simulink model "case2mod"  (Simulink 7.7)
settings: Solver=FixedStepDiscrete  StartTime=0.0  StopTime=25000  FixedStep=1  RelTol=1e-3
libraries: SimpleModeling x38
settings Model: Creator=iris  LastModifiedBy=iris
settings DataIOCC: SaveFormat=StructureWithTime
settings OptimizationCC: BlockReduction=off  ConditionallyExecuteInputs=off

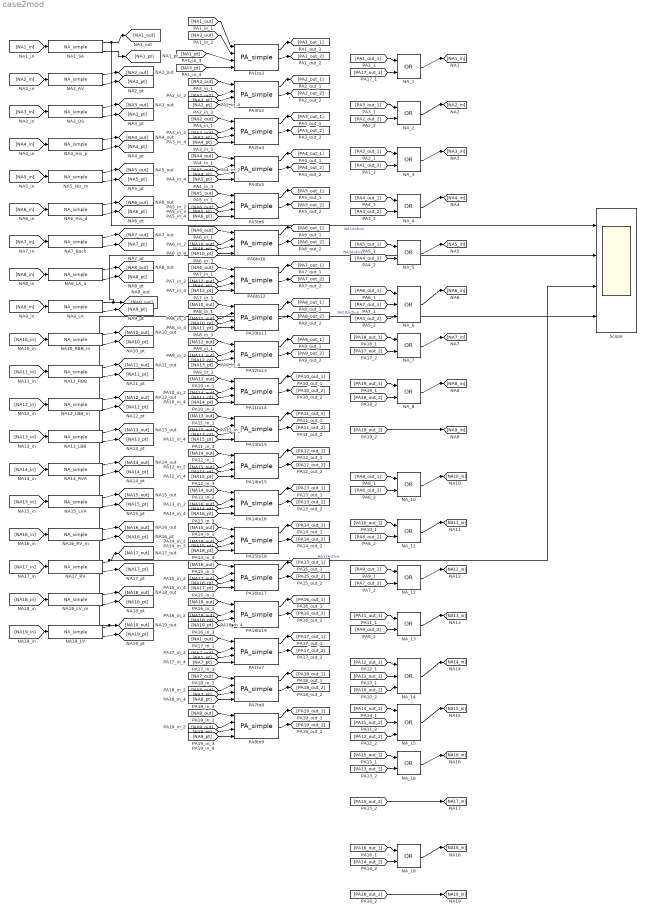
== system case2mod ==
  NA10_RBB_m : SimpleModeling/NA_simple  SystemSampleTime=-1  TERP_defs=320  TRRP_def=120  Trest_def=9999  TERP_s=320  TRRP_s=120  Trest_s=9999  Terp_min=150  Terp_max=300
  NA11_RBB : SimpleModeling/NA_simple  SystemSampleTime=-1  TERP_defs=320  TRRP_def=120  Trest_def=9999  TERP_s=320  TRRP_s=120  Trest_s=9999  Terp_min=150  Terp_max=300
  NA12_LBB_m : SimpleModeling/NA_simple  SystemSampleTime=-1  TERP_defs=320  TRRP_def=120  Trest_def=9999  TERP_s=320  TRRP_s=120  Trest_s=9999  Terp_min=150  Terp_max=300
  NA13_LBB : SimpleModeling/NA_simple  SystemSampleTime=-1  TERP_defs=320  TRRP_def=120  Trest_def=9999  TERP_s=320  TRRP_s=120  Trest_s=9999  Terp_min=150  Terp_max=300
  NA14_RVA : SimpleModeling/NA_simple  SystemSampleTime=-1  TERP_defs=320  TRRP_def=120  Trest_def=9999  TERP_s=320  TRRP_s=120  Trest_s=9999  Terp_min=150  Terp_max=300
  NA15_LVA : SimpleModeling/NA_simple  SystemSampleTime=-1  TERP_defs=320  TRRP_def=120  Trest_def=9999  TERP_s=320  TRRP_s=120  Trest_s=9999  Terp_min=150  Terp_max=300
  NA16_RV_m : SimpleModeling/NA_simple  SystemSampleTime=-1  TERP_defs=320  TRRP_def=120  Trest_def=9999  TERP_s=320  TRRP_s=120  Trest_s=9999  Terp_min=150  Terp_max=300
  NA17_RV : SimpleModeling/NA_simple  SystemSampleTime=-1  TERP_defs=320  TRRP_def=120  Trest_def=9999  TERP_s=320  TRRP_s=120  Trest_s=9999  Terp_min=150  Terp_max=300
  NA18_LV_m : SimpleModeling/NA_simple  SystemSampleTime=-1  TERP_defs=320  TRRP_def=120  Trest_def=9999  TERP_s=320  TRRP_s=120  Trest_s=9999  Terp_min=150  Terp_max=300
  NA19_LV : SimpleModeling/NA_simple  SystemSampleTime=-1  TERP_defs=320  TRRP_def=120  Trest_def=9999  TERP_s=320  TRRP_s=120  Trest_s=9999  Terp_min=150  Terp_max=300
  NA1_SA : SimpleModeling/NA_simple  SystemSampleTime=-1  TERP_defs=320  TRRP_def=100  Trest_def=800  TERP_s=320  TRRP_s=100  Trest_s=800  Terp_min=150  Terp_max=300
  NA2_AV : SimpleModeling/NA_simple  SystemSampleTime=-1  TERP_defs=320  TRRP_def=350  Trest_def=9999  TERP_s=320  TRRP_s=350  Trest_s=9999  Terp_min=800  Terp_max=350
  NA3_OS : SimpleModeling/NA_simple  SystemSampleTime=-1  TERP_defs=320  TRRP_def=120  Trest_def=9999  TERP_s=320  TRRP_s=120  Trest_s=9999  Terp_min=150  Terp_max=300
  NA4_His_p : SimpleModeling/NA_simple  SystemSampleTime=-1  TERP_defs=320  TRRP_def=120  Trest_def=9999  TERP_s=320  TRRP_s=120  Trest_s=9999  Terp_min=150  Terp_max=300
  NA5_His_m : SimpleModeling/NA_simple  SystemSampleTime=-1  TERP_defs=320  TRRP_def=120  Trest_def=9999  TERP_s=320  TRRP_s=120  Trest_s=9999  Terp_min=150  Terp_max=300
  NA6_His_d : SimpleModeling/NA_simple  SystemSampleTime=-1  TERP_defs=320  TRRP_def=120  Trest_def=9999  TERP_s=320  TRRP_s=120  Trest_s=9999  Terp_min=150  Terp_max=300
  NA7_Bach : SimpleModeling/NA_simple  SystemSampleTime=-1  TERP_defs=320  TRRP_def=120  Trest_def=9999  TERP_s=320  TRRP_s=120  Trest_s=9999  Terp_min=150  Terp_max=300
  NA8_LA_a : SimpleModeling/NA_simple  SystemSampleTime=-1  TERP_defs=320  TRRP_def=120  Trest_def=9999  TERP_s=320  TRRP_s=120  Trest_s=9999  Terp_min=150  Terp_max=300
  NA9_LA : SimpleModeling/NA_simple  SystemSampleTime=-1  TERP_defs=320  TRRP_def=120  Trest_def=9999  TERP_s=320  TRRP_s=120  Trest_s=9999  Terp_min=150  Terp_max=300
  NA_{1..5,7..8,10..13,16,18} (13 alike) : Logic  Operator=OR  AllPortsSameDT=off  OutDataTypeStr=boolean
  NA_14 : Logic  Operator=OR  Inputs=3  AllPortsSameDT=off  OutDataTypeStr=boolean
  NA_15 : Logic  Operator=OR  Inputs=3  AllPortsSameDT=off  OutDataTypeStr=boolean
  NA_6 : Logic  Operator=OR  Inputs=3  AllPortsSameDT=off  OutDataTypeStr=boolean
  PA10to11 : SimpleModeling/PA_simple  SystemSampleTime=-1  min_path_par=10  bck_param=43  forw_param=43
  PA11to14 : SimpleModeling/PA_simple  SystemSampleTime=-1  min_path_par=9  bck_param=9  forw_param=9
  PA12to13 : SimpleModeling/PA_simple  SystemSampleTime=-1  min_path_par=38  bck_param=38  forw_param=38
  PA13to15 : SimpleModeling/PA_simple  SystemSampleTime=-1  min_path_par=9  bck_param=10  forw_param=10
  PA14to15 : SimpleModeling/PA_simple  SystemSampleTime=-1  min_path_par=17  bck_param=18  forw_param=18
  PA14to16 : SimpleModeling/PA_simple  SystemSampleTime=-1  min_path_par=58  bck_param=58  forw_param=58
  PA15to18 : SimpleModeling/PA_simple  SystemSampleTime=-1  min_path_par=46  bck_param=46  forw_param=46
  PA16to17 : SimpleModeling/PA_simple  SystemSampleTime=-1  min_path_par=53  bck_param=53  forw_param=53
  PA18to19 : SimpleModeling/PA_simple  SystemSampleTime=-1  min_path_par=39  bck_param=40  forw_param=40
  PA1to3 : SimpleModeling/PA_simple  SystemSampleTime=-1  min_path_par=22  bck_param=22  forw_param=22
  PA1to7 : SimpleModeling/PA_simple  SystemSampleTime=-1  min_path_par=60  bck_param=60  forw_param=60
  PA2to4 : SimpleModeling/PA_simple  SystemSampleTime=-1  min_path_par=93  bck_param=3000  forw_param=47
  PA3to2 : SimpleModeling/PA_simple  SystemSampleTime=-1  min_path_par=24  bck_param=24  forw_param=24
  PA4to5 : SimpleModeling/PA_simple  SystemSampleTime=-1  min_path_par=16  bck_param=16  forw_param=16
  PA5to6 : SimpleModeling/PA_simple  SystemSampleTime=-1  min_path_par=20  bck_param=20  forw_param=20
  PA6to10 : SimpleModeling/PA_simple  SystemSampleTime=-1  min_path_par=10  bck_param=36  forw_param=36
  PA6to12 : SimpleModeling/PA_simple  SystemSampleTime=-1  min_path_par=37  bck_param=38  forw_param=38
  PA7to8 : SimpleModeling/PA_simple  SystemSampleTime=-1  min_path_par=34  bck_param=34  forw_param=34
  PA8to9 : SimpleModeling/PA_simple  SystemSampleTime=-1  min_path_par=17  bck_param=18  forw_param=18
  Scope : Scope  NumInputPorts=4
      settings: TimeRange=25000  YMin=0~0~0~0  YMax=1~1~1~1
  wires:
  NA1_SA/1 -> [NA1_out], Scope/1  "NA1Active"
  NA1_SA/3 -> [NA1_pt]
  [NA1_in] -> NA1_SA/1
  [PA1_out_1] -> NA_1/1
  [PA17_out_1] -> NA_1/2
  NA_1/1 -> [NA1_in]
  NA2_AV/1 -> [NA2_out]
  NA2_AV/3 -> [NA2_pt]
  [NA2_in] -> NA2_AV/1
  [PA3_out_1] -> NA_2/1
  [PA2_out_2] -> NA_2/2
  NA_2/1 -> [NA2_in]
  NA3_OS/1 -> [NA3_out]
  NA3_OS/3 -> [NA3_pt]
  [NA3_in] -> NA3_OS/1
  [PA2_out_1] -> NA_3/1
  [PA1_out_2] -> NA_3/2
  NA_3/1 -> [NA3_in]
  NA4_His_p/1 -> [NA4_out]
  NA4_His_p/3 -> [NA4_pt]
  [NA4_in] -> NA4_His_p/1
  [PA4_out_1] -> NA_4/1
  [PA3_out_2] -> NA_4/2
  NA_4/1 -> [NA4_in]
  NA5_His_m/1 -> [NA5_out]
  NA5_His_m/3 -> [NA5_pt]
  [NA5_in] -> NA5_His_m/1
  [PA5_out_1] -> NA_5/1
  [PA4_out_2] -> NA_5/2
  NA_5/1 -> [NA5_in]
  NA6_His_d/1 -> [NA6_out]
  NA6_His_d/3 -> [NA6_pt]
  [NA6_in] -> NA6_His_d/1
  [PA6_out_1] -> NA_6/1
  [PA7_out_1] -> NA_6/2
  [PA5_out_2] -> NA_6/3
  NA_6/1 -> [NA6_in]
  NA7_Bach/1 -> [NA7_out]
  NA7_Bach/3 -> [NA7_pt]
  [NA7_in] -> NA7_Bach/1
  [PA18_out_1] -> NA_7/1
  [PA17_out_2] -> NA_7/2
  NA_7/1 -> [NA7_in]
  NA8_LA_a/1 -> [NA8_out]
  NA8_LA_a/3 -> [NA8_pt]
  [NA8_in] -> NA8_LA_a/1
  [PA19_out_1] -> NA_8/1
  [PA18_out_2] -> NA_8/2
  NA_8/1 -> [NA8_in]
  NA9_LA/1 -> [NA9_out], Scope/2  "NA9Active"
  NA9_LA/3 -> [NA9_pt]
  [NA9_in] -> NA9_LA/1
  [PA19_out_2] -> [NA9_in]
  NA10_RBB_m/1 -> [NA10_out]
  NA10_RBB_m/3 -> [NA10_pt]
  [NA10_in] -> NA10_RBB_m/1
  [PA8_out_1] -> NA_10/1
  [PA6_out_2] -> NA_10/2
  NA_10/1 -> [NA10_in]
  NA11_RBB/1 -> [NA11_out]
  NA11_RBB/3 -> [NA11_pt]
  [NA11_in] -> NA11_RBB/1
  [PA10_out_1] -> NA_11/1
  [PA8_out_2] -> NA_11/2
  NA_11/1 -> [NA11_in]
  NA12_LBB_m/1 -> [NA12_out]
  NA12_LBB_m/3 -> [NA12_pt]
  [NA12_in] -> NA12_LBB_m/1
  [PA9_out_1] -> NA_12/1
  [PA7_out_2] -> NA_12/2
  NA_12/1 -> [NA12_in]
  NA13_LBB/1 -> [NA13_out]
  NA13_LBB/3 -> [NA13_pt]
  [NA13_in] -> NA13_LBB/1
  [PA11_out_1] -> NA_13/1
  [PA9_out_2] -> NA_13/2
  NA_13/1 -> [NA13_in]
  NA14_RVA/1 -> [NA14_out]
  NA14_RVA/3 -> [NA14_pt]
  [NA14_in] -> NA14_RVA/1
  [PA12_out_1] -> NA_14/1
  [PA13_out_1] -> NA_14/2
  [PA10_out_2] -> NA_14/3
  NA_14/1 -> [NA14_in]
  NA15_LVA/1 -> [NA15_out]
  NA15_LVA/3 -> [NA15_pt]
  [NA15_in] -> NA15_LVA/1
  [PA14_out_1] -> NA_15/1
  [PA11_out_2] -> NA_15/2
  [PA12_out_2] -> NA_15/3
  NA_15/1 -> [NA15_in]
  NA16_RV_m/1 -> [NA16_out]
  NA16_RV_m/3 -> [NA16_pt]
  [NA16_in] -> NA16_RV_m/1
  [PA15_out_1] -> NA_16/1
  [PA13_out_2] -> NA_16/2
  NA_16/1 -> [NA16_in]
  NA17_RV/1 -> [NA17_out], Scope/3  "NA17Active"
  NA17_RV/3 -> [NA17_pt]
  [NA17_in] -> NA17_RV/1
  [PA15_out_2] -> [NA17_in]
  NA18_LV_m/1 -> [NA18_out]
  NA18_LV_m/3 -> [NA18_pt]
  [NA18_in] -> NA18_LV_m/1
  [PA16_out_1] -> NA_18/1
  [PA14_out_2] -> NA_18/2
  NA_18/1 -> [NA18_in]
  NA19_LV/1 -> [NA19_out], Scope/4  "NA19Active"
  NA19_LV/3 -> [NA19_pt]
  [NA19_in] -> NA19_LV/1
  [PA16_out_2] -> [NA19_in]
  PA1to3/1 -> [PA1_out_1]
  PA1to3/2 -> [PA1_out_2]
  [NA1_out] -> PA1to3/1
  [NA3_out] -> PA1to3/2
  [NA1_pt] -> PA1to3/3
  [NA3_pt] -> PA1to3/4
  PA3to2/1 -> [PA2_out_1]
  PA3to2/2 -> [PA2_out_2]
  [NA3_out] -> PA3to2/1
  [NA2_out] -> PA3to2/2
  [NA3_pt] -> PA3to2/3
  [NA2_pt] -> PA3to2/4
  PA2to4/1 -> [PA3_out_1]
  PA2to4/2 -> [PA3_out_2]
  [NA2_out] -> PA2to4/1
  [NA4_out] -> PA2to4/2
  [NA2_pt] -> PA2to4/3
  [NA4_pt] -> PA2to4/4
  PA4to5/1 -> [PA4_out_1]
  PA4to5/2 -> [PA4_out_2]
  [NA4_out] -> PA4to5/1
  [NA5_out] -> PA4to5/2
  [NA4_pt] -> PA4to5/3
  [NA5_pt] -> PA4to5/4
  PA5to6/1 -> [PA5_out_1]
  PA5to6/2 -> [PA5_out_2]
  [NA5_out] -> PA5to6/1
  [NA6_out] -> PA5to6/2
  [NA5_pt] -> PA5to6/3
  [NA6_pt] -> PA5to6/4
  PA6to10/1 -> [PA6_out_1]
  PA6to10/2 -> [PA6_out_2]
  [NA6_out] -> PA6to10/1
  [NA10_out] -> PA6to10/2
  [NA6_pt] -> PA6to10/3
  [NA10_pt] -> PA6to10/4
  PA6to12/1 -> [PA7_out_1]
  PA6to12/2 -> [PA7_out_2]
  [NA6_out] -> PA6to12/1
  [NA12_out] -> PA6to12/2
  [NA6_pt] -> PA6to12/3
  [NA12_pt] -> PA6to12/4
  PA10to11/1 -> [PA8_out_1]
  PA10to11/2 -> [PA8_out_2]
  [NA10_out] -> PA10to11/1
  [NA11_out] -> PA10to11/2
  [NA10_pt] -> PA10to11/3
  [NA11_pt] -> PA10to11/4
  PA12to13/1 -> [PA9_out_1]
  PA12to13/2 -> [PA9_out_2]
  [NA12_out] -> PA12to13/1
  [NA13_out] -> PA12to13/2
  [NA12_pt] -> PA12to13/3
  [NA13_pt] -> PA12to13/4
  PA11to14/1 -> [PA10_out_1]
  PA11to14/2 -> [PA10_out_2]
  [NA11_out] -> PA11to14/1
  [NA14_out] -> PA11to14/2
  [NA11_pt] -> PA11to14/3
  [NA14_pt] -> PA11to14/4
  PA13to15/1 -> [PA11_out_1]
  PA13to15/2 -> [PA11_out_2]
  [NA13_out] -> PA13to15/1
  [NA15_out] -> PA13to15/2
  [NA13_pt] -> PA13to15/3
  [NA15_pt] -> PA13to15/4
  PA14to15/1 -> [PA12_out_1]
  PA14to15/2 -> [PA12_out_2]
  [NA14_out] -> PA14to15/1
  [NA15_out] -> PA14to15/2
  [NA14_pt] -> PA14to15/3
  [NA15_pt] -> PA14to15/4
  PA14to16/1 -> [PA13_out_1]
  PA14to16/2 -> [PA13_out_2]
  [NA14_out] -> PA14to16/1
  [NA16_out] -> PA14to16/2
  [NA14_pt] -> PA14to16/3
  [NA16_pt] -> PA14to16/4
  PA15to18/1 -> [PA14_out_1]
  PA15to18/2 -> [PA14_out_2]
  [NA15_out] -> PA15to18/1
  [NA18_out] -> PA15to18/2
  [NA15_pt] -> PA15to18/3
  [NA18_pt] -> PA15to18/4
  PA16to17/1 -> [PA15_out_1]
  PA16to17/2 -> [PA15_out_2]
  [NA16_out] -> PA16to17/1
  [NA17_out] -> PA16to17/2
  [NA16_pt] -> PA16to17/3
  [NA17_pt] -> PA16to17/4
  PA18to19/1 -> [PA16_out_1]
  PA18to19/2 -> [PA16_out_2]
  [NA18_out] -> PA18to19/1
  [NA19_out] -> PA18to19/2
  [NA18_pt] -> PA18to19/3
  [NA19_pt] -> PA18to19/4
  PA1to7/1 -> [PA17_out_1]
  PA1to7/2 -> [PA17_out_2]
  [NA1_out] -> PA1to7/1
  [NA7_out] -> PA1to7/2
  [NA1_pt] -> PA1to7/3
  [NA7_pt] -> PA1to7/4
  PA7to8/1 -> [PA18_out_1]
  PA7to8/2 -> [PA18_out_2]
  [NA7_out] -> PA7to8/1
  [NA8_out] -> PA7to8/2
  [NA7_pt] -> PA7to8/3
  [NA8_pt] -> PA7to8/4
  PA8to9/1 -> [PA19_out_1]
  PA8to9/2 -> [PA19_out_2]
  [NA8_out] -> PA8to9/1
  [NA9_out] -> PA8to9/2
  [NA8_pt] -> PA8to9/3
  [NA9_pt] -> PA8to9/4
